simulink library "INP_IMU_PrepAngRat2"  (R2024b)
settings: Solver=VariableStepAuto  StartTime=0.0  StopTime=10.0  RelTol=1e-3
undefined symbols (not defined in the file): INP_c_TiSample_s, INP_IMU_p_AngRatPitchVehOfs_radps, INP_IMU_p_AngRatPitchVehSca_na, INP_IMU_p_AngRatRollVehOfs_radps, INP_IMU_p_AngRatRollVehSca_na, INP_IMU_p_AngRatYawVehOfs_radps, INP_IMU_p_AngRatYawVehSca_na, INP_p_TiTau_s
libraries: VUT_lib x3
settings Model: Creator=blatak  LastModifiedBy=blatak
settings RTWCC: GPUComputeCapability=3.5

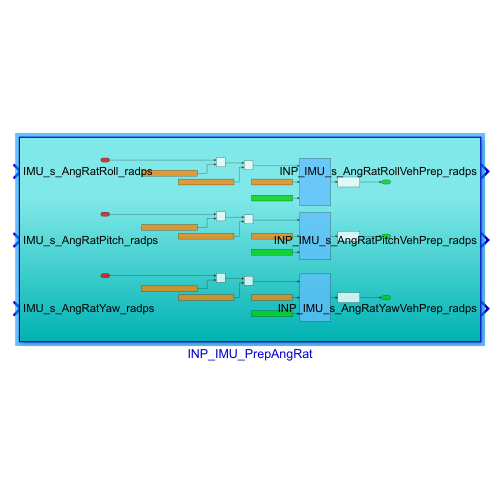
[thumbnail: Simulink's stored preview of the top-level diagram]
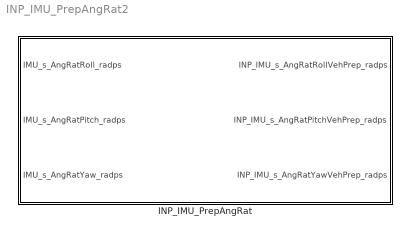
== system INP_IMU_PrepAngRat2 ==
  INP_IMU_PrepAngRat : Subsystem  Description=Block transfers the value from electric quantitty to physical one (if needed), afterthat low pass filter is applied.

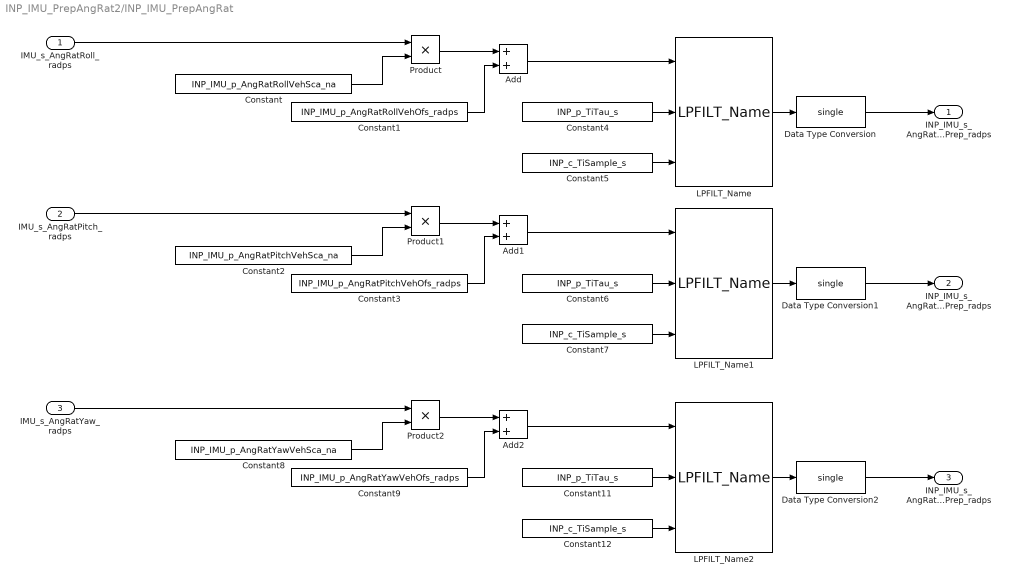
== system INP_IMU_PrepAngRat2/INP_IMU_PrepAngRat ==
  IMU_s_AngRatRoll_radps : Inport  Description=IMU Angular roll velocity - raw measured value from sensor
  IMU_s_AngRatPitch_radps : Inport  Description=IMU Angular pitch velocity - raw measured value from sensor  Port=2
  IMU_s_AngRatYaw_radps : Inport  Description=IMU Angular yaw velocity - raw measured value from sensor  Port=3
  Add : Sum
  Add1 : Sum
  Add2 : Sum
  Constant : Constant  Description=Scaling coefficient to recalculate the electric quantity to the physical one - roll velocity  Value=INP_IMU_p_AngRatRollVehSca_na
  Constant1 : Constant  Description=Offset to recalculate the electric quantity to the physical one - roll velocity  Value=INP_IMU_p_AngRatRollVehOfs_radps
  Constant11 : Constant  Value=INP_p_TiTau_s
  Constant12 : Constant  Value=INP_c_TiSample_s
  Constant2 : Constant  Description=Scaling coefficient to recalculate the electric quantity to the physical one - pitch velocity  Value=INP_IMU_p_AngRatPitchVehSca_na
  Constant3 : Constant  Description=Offset to recalculate the electric quantity to the physical one - pitch velocity  Value=INP_IMU_p_AngRatPitchVehOfs_radps
  Constant4 : Constant  Value=INP_p_TiTau_s
  Constant5 : Constant  Value=INP_c_TiSample_s
  Constant6 : Constant  Value=INP_p_TiTau_s
  Constant7 : Constant  Value=INP_c_TiSample_s
  Constant8 : Constant  Description=Scaling coefficient to recalculate the electric quantity to the physical one - yaw velocity  Value=INP_IMU_p_AngRatYawVehSca_na
  Constant9 : Constant  Description=Offset to recalculate the electric quantity to the physical one - yaw velocity  Value=INP_IMU_p_AngRatYawVehOfs_radps
  Data Type Conversion : DataTypeConversion  OutDataTypeStr=single  SaturateOnIntegerOverflow=off  RndMeth=Floor
  Data Type Conversion1 : DataTypeConversion  OutDataTypeStr=single  SaturateOnIntegerOverflow=off  RndMeth=Floor
  Data Type Conversion2 : DataTypeConversion  OutDataTypeStr=single  SaturateOnIntegerOverflow=off  RndMeth=Floor
  LPFILT_Name : VUT_lib/LPFILT_Name  SystemSampleTime=-1  VariantActivationTime=update diagram  AllowFlexibleInterface=on  Latency=0  AutoFrameSizeCalculation=off
  LPFILT_Name1 : VUT_lib/LPFILT_Name  SystemSampleTime=-1  VariantActivationTime=update diagram  AllowFlexibleInterface=on  Latency=0  AutoFrameSizeCalculation=off
  LPFILT_Name2 : VUT_lib/LPFILT_Name  SystemSampleTime=-1  VariantActivationTime=update diagram  AllowFlexibleInterface=on  Latency=0  AutoFrameSizeCalculation=off
  Product : Product
  Product1 : Product
  Product2 : Product
  INP_IMU_s_AngRatRollVehPrep_radps : Outport  Description=IMU Angular roll velocity - prepared - scale, offset, filtering
  INP_IMU_s_AngRatPitchVehPrep_radps : Outport  Description=IMU Angular pitch velocity - prepared - scale, offset, filtering  Port=2
  INP_IMU_s_AngRatYawVehPrep_radps : Outport  Description=IMU Angular yaw velocity - prepared - scale, offset, filtering  Port=3
  wires:
  IMU_s_AngRatPitch_radps/1 -> Product1/1
  Product1/1 -> Add1/1
  IMU_s_AngRatRoll_radps/1 -> Product/1
  Constant5/1 -> LPFILT_Name/3
  Constant9/1 -> Add2/2
  Add2/1 -> LPFILT_Name2/1
  LPFILT_Name1/1 -> Data Type Conversion1/1
  Constant/1 -> Product/2
  Constant12/1 -> LPFILT_Name2/3
  Product2/1 -> Add2/1
  LPFILT_Name/1 -> Data Type Conversion/1
  IMU_s_AngRatYaw_radps/1 -> Product2/1
  Constant7/1 -> LPFILT_Name1/3
  Constant6/1 -> LPFILT_Name1/2
  Add/1 -> LPFILT_Name/1
  Product/1 -> Add/1
  LPFILT_Name2/1 -> Data Type Conversion2/1
  Constant3/1 -> Add1/2
  Constant8/1 -> Product2/2
  Constant11/1 -> LPFILT_Name2/2
  Constant1/1 -> Add/2
  Constant4/1 -> LPFILT_Name/2
  Constant2/1 -> Product1/2
  Add1/1 -> LPFILT_Name1/1
  Data Type Conversion/1 -> INP_IMU_s_AngRatRollVehPrep_radps/1
  Data Type Conversion1/1 -> INP_IMU_s_AngRatPitchVehPrep_radps/1
  Data Type Conversion2/1 -> INP_IMU_s_AngRatYawVehPrep_radps/1
